simulink model "batterymodelsimu"  (R2022b)
settings: Solver=VariableStepAuto  StartTime=0.0  StopTime=10.0  RelTol=1e-3
InitFcn:
  | batterymodelsimu
undefined symbols (not defined in the file or in its folder): A, B, D, Ki1, Ki2, Kp, new_ai, new_bi, x
settings Model: Creator=12159  LastModifiedBy=12159

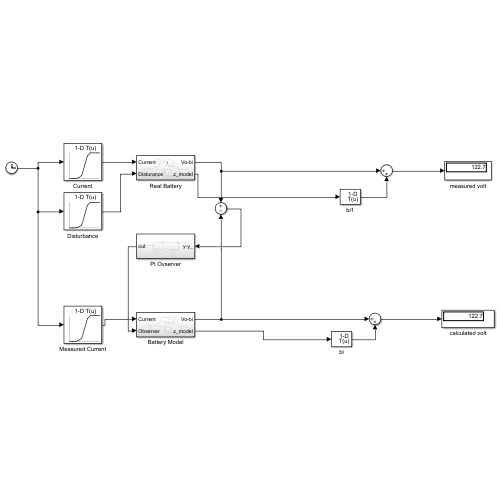
[thumbnail: Simulink's stored preview of the top-level diagram]
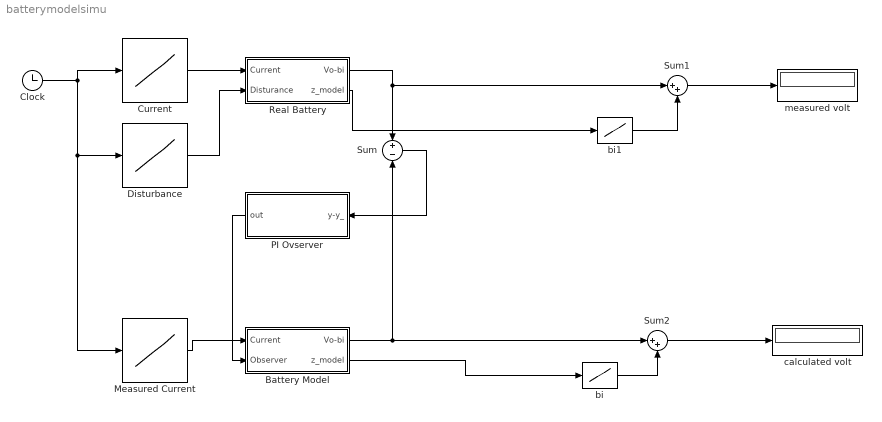
== system batterymodelsimu ==
  Battery Model : Subsystem
  Clock : Clock
  Current : Lookup_n-D  NumberOfTableDimensions=1  BreakpointsForDimension1=[-5:5]  Table=tanh([-5:5])  InternalRulePriority=Speed  RndMeth=Simplest
  Disturbance : Lookup_n-D  NumberOfTableDimensions=1  BreakpointsForDimension1=[-5:5]  Table=tanh([-5:5])  InternalRulePriority=Speed  RndMeth=Simplest
  Measured Current : Lookup_n-D  NumberOfTableDimensions=1  BreakpointsForDimension1=[-5:5]  Table=tanh([-5:5])  InternalRulePriority=Speed  RndMeth=Simplest
  PI Ovserver : Subsystem
  Real Battery : Subsystem
  Sum : Sum  Inputs=+-
  Sum1 : Sum  Inputs=|++
  Sum2 : Sum  Inputs=|++
  bi : Lookup_n-D  NumberOfTableDimensions=1  BreakpointsForDimension1=x  Table=new_bi  InternalRulePriority=Speed  RndMeth=Simplest
  bi1 : Lookup_n-D  NumberOfTableDimensions=1  BreakpointsForDimension1=x  Table=new_bi  InternalRulePriority=Speed  RndMeth=Simplest
  calculated volt : Display
  measured volt : Display
  wires:
  Clock/1 -> Measured Current/1, Disturbance/1, Current/1
  Current/1 -> Real Battery/1(Current)
  Disturbance/1 -> Real Battery/2(Disturance)
  Measured Current/1 -> Battery Model/1(Current)
  Sum/1 -> PI Ovserver/1(y-y_)
  Real Battery/1(Vo-bi) -> Sum/1, Sum1/1
  PI Ovserver/1(out) -> Battery Model/2(Observer)
  Battery Model/1(Vo-bi) -> Sum/2, Sum2/1
  Battery Model/2(z_model) -> bi/1
  bi/1 -> Sum2/2
  Sum2/1 -> calculated volt/1
  Real Battery/2(z_model) -> bi1/1
  bi1/1 -> Sum1/2
  Sum1/1 -> measured volt/1

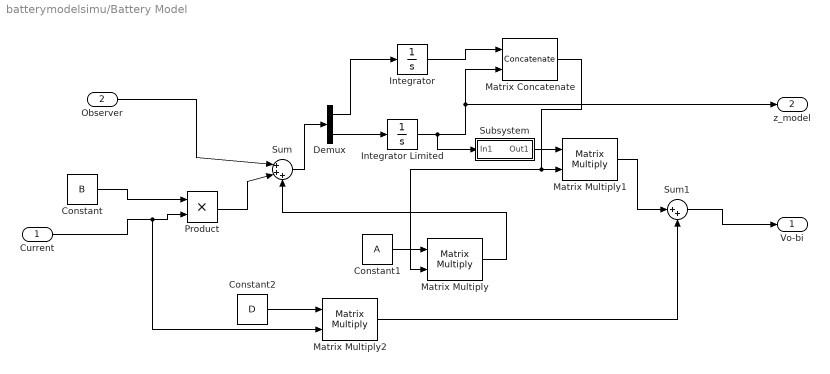
== system batterymodelsimu/Battery Model ==
  Current : Inport
  Observer : Inport  Port=2
  Constant : Constant  Value=B
  Constant1 : Constant  Value=A
  Constant2 : Constant  Value=D
  Demux : Demux  Outputs=2
  Integrator : Integrator
  Integrator Limited : Integrator  LimitOutput=on  UpperSaturationLimit=100  LowerSaturationLimit=0
  Matrix Concatenate : Concatenate  Mode=Multidimensional array
  Matrix Multiply : Product  Multiplication=Matrix(*)
  Matrix Multiply1 : Product  Multiplication=Matrix(*)
  Matrix Multiply2 : Product  Multiplication=Matrix(*)
  Product : Product
  Subsystem : Subsystem
  Sum : Sum  Inputs=|+++
  Sum1 : Sum  Inputs=|++
  Vo-bi : Outport
  z_model : Outport  Port=2
  wires:
  Constant/1 -> Product/1
  Current/1 -> Product/2, Matrix Multiply2/2
  Constant1/1 -> Matrix Multiply/1
  Observer/1 -> Sum/1
  Product/1 -> Sum/2
  Matrix Multiply/1 -> Sum/3
  Sum/1 -> Demux/1
  Constant2/1 -> Matrix Multiply2/1
  Demux/1 -> Integrator/1
  Demux/2 -> Integrator Limited/1
  Integrator/1 -> Matrix Concatenate/1
  Integrator Limited/1 -> Subsystem/1(In1), Matrix Concatenate/2, z_model/1
  Matrix Concatenate/1 -> Matrix Multiply/2, Matrix Multiply1/2
  Matrix Multiply1/1 -> Sum1/1
  Matrix Multiply2/1 -> Sum1/2
  Sum1/1 -> Vo-bi/1
  Subsystem/1(Out1) -> Matrix Multiply1/1

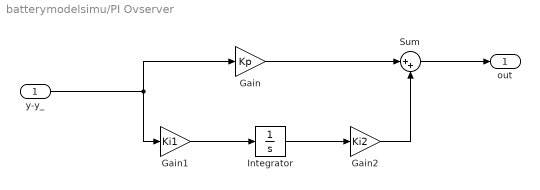
== system batterymodelsimu/PI Ovserver ==
  y-y_ : Inport
  Gain : Gain  Gain=Kp
  Gain1 : Gain  Gain=Ki1
  Gain2 : Gain  Gain=Ki2
  Integrator : Integrator
  Sum : Sum  Inputs=|++
  out : Outport
  wires:
  y-y_/1 -> Gain1/1, Gain/1
  Gain/1 -> Sum/1
  Gain1/1 -> Integrator/1
  Integrator/1 -> Gain2/1
  Gain2/1 -> Sum/2
  Sum/1 -> out/1

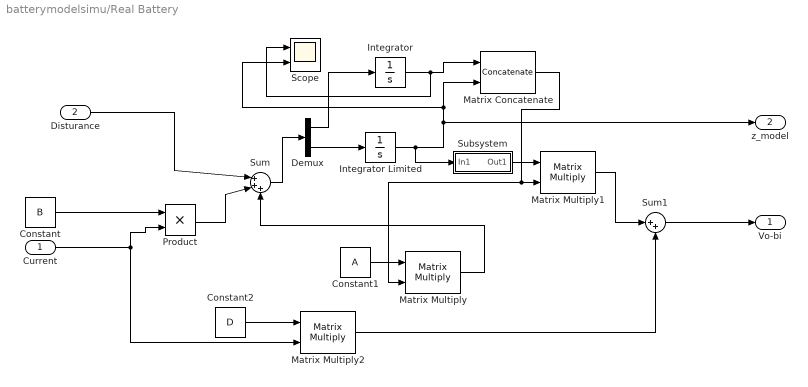
== system batterymodelsimu/Real Battery ==
  Current : Inport
  Disturance : Inport  Port=2
  Constant : Constant  Value=B
  Constant1 : Constant  Value=A
  Constant2 : Constant  Value=D
  Demux : Demux  Outputs=2
  Integrator : Integrator
  Integrator Limited : Integrator  LimitOutput=on  UpperSaturationLimit=100  LowerSaturationLimit=0
  Matrix Concatenate : Concatenate  Mode=Multidimensional array
  Matrix Multiply : Product  Multiplication=Matrix(*)
  Matrix Multiply1 : Product  Multiplication=Matrix(*)
  Matrix Multiply2 : Product  Multiplication=Matrix(*)
  Product : Product
  Scope : Scope  NumInputPorts=2
  Subsystem : Subsystem
  Sum : Sum  Inputs=|+++
  Sum1 : Sum  Inputs=|++
  Vo-bi : Outport
  z_model : Outport  Port=2
  wires:
  Subsystem/1(Out1) -> Matrix Multiply1/1
  Sum1/1 -> Vo-bi/1
  Constant2/1 -> Matrix Multiply2/1
  Matrix Multiply/1 -> Sum/3
  Constant1/1 -> Matrix Multiply/1
  Demux/2 -> Integrator Limited/1
  Matrix Multiply1/1 -> Sum1/1
  Disturance/1 -> Sum/1
  Integrator Limited/1 -> Subsystem/1(In1), z_model/1, Scope/2, Matrix Concatenate/2
  Current/1 -> Product/2, Matrix Multiply2/2
  Demux/1 -> Integrator/1
  Integrator/1 -> Scope/1, Matrix Concatenate/1
  Product/1 -> Sum/2
  Sum/1 -> Demux/1
  Matrix Multiply2/1 -> Sum1/2
  Constant/1 -> Product/1
  Matrix Concatenate/1 -> Matrix Multiply/2, Matrix Multiply1/2

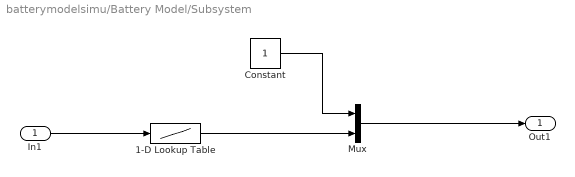
== system batterymodelsimu/Battery Model/Subsystem ==
  In1 : Inport
  1-D Lookup Table : Lookup_n-D  NumberOfTableDimensions=1  BreakpointsForDimension1=x  Table=new_ai  InternalRulePriority=Speed  RndMeth=Simplest
  Constant : Constant
  Mux : Mux  Inputs=2
  Out1 : Outport
  wires:
  In1/1 -> 1-D Lookup Table/1
  Constant/1 -> Mux/1
  1-D Lookup Table/1 -> Mux/2
  Mux/1 -> Out1/1

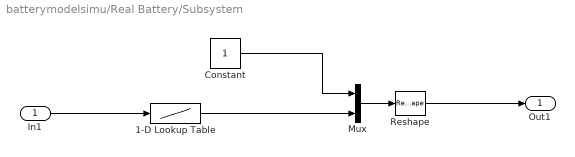
== system batterymodelsimu/Real Battery/Subsystem ==
  In1 : Inport
  1-D Lookup Table : Lookup_n-D  NumberOfTableDimensions=1  BreakpointsForDimension1=x  Table=new_ai  InternalRulePriority=Speed  RndMeth=Simplest
  Constant : Constant
  Mux : Mux  Inputs=2
  Reshape : Reshape  OutputDimensionality=Customize  OutputDimensions=[1,2]
  Out1 : Outport
  wires:
  In1/1 -> 1-D Lookup Table/1
  Constant/1 -> Mux/1
  1-D Lookup Table/1 -> Mux/2
  Mux/1 -> Reshape/1
  Reshape/1 -> Out1/1
